simulink model "Discrete_vs_continous"  (R2013a)
settings: Solver=ode45  StartTime=0.0  StopTime=0.1  FixedStep=0.000001  RelTol=1e-3
settings Model: Creator=Max Simmonds  LastModifiedBy=Max Simmonds
settings DebuggingCC: SolverPrmCheckMsg=none

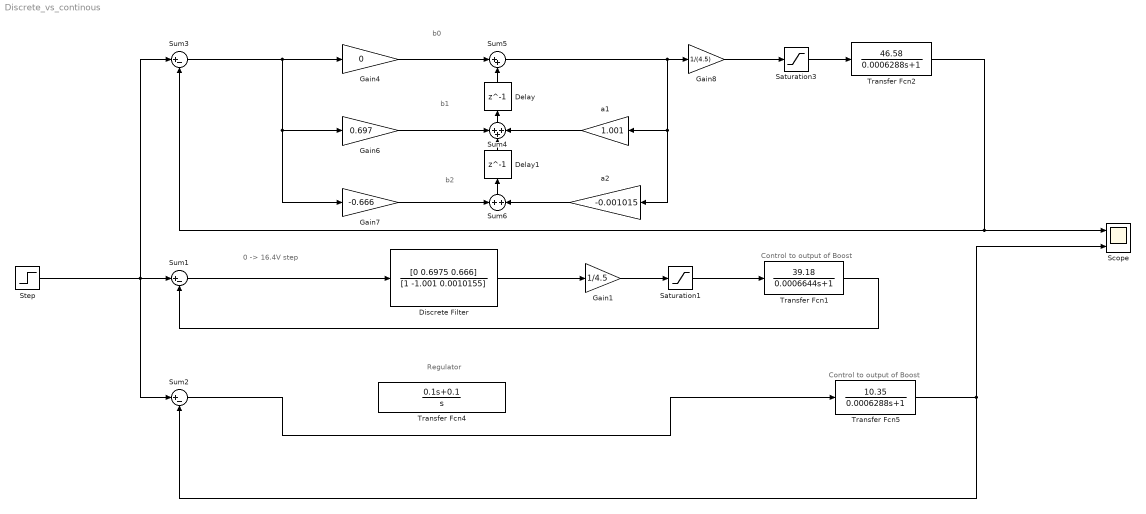
== system Discrete_vs_continous ==
  note: b2
  note: b1
  note: b0
  note: 0 -> 16.4V step
  note: Control to output of Boost
  note: Regulator
  note: Control to output of Boost
  Delay : Delay  DelayLength=1  InitialCondition=0  SampleTime=4e-5
  Delay1 : Delay  DelayLength=1  InitialCondition=0  SampleTime=4e-5
  Discrete Filter : DiscreteFilter  Numerator=[0 0.6975 0.666]  Denominator=[1 -1.001 0.0010155]  SampleTime=4e-5
  Gain1 : Gain  Gain=1/4.5
  Gain4 : Gain  Gain=0  SampleTime=4e-5
  Gain6 : Gain  Gain=0.697  SampleTime=4e-5
  Gain7 : Gain  Gain=-0.666  SampleTime=4e-5
  Gain8 : Gain  Gain=1/(4.5)  SampleTime=4e-5
  Saturation1 : Saturate  UpperLimit=0.9  LowerLimit=0.1
  Saturation3 : Saturate  UpperLimit=0.7  LowerLimit=0.1
  Scope : Scope  NumInputPorts=2
      settings: TimeRange=0.003173749327595482  YMin=15.58~0.334478  YMax=17.22~0.369686
  Step : Step  Time=0.01  Before=0.1  After=16.4  SampleTime=4e-5
  Sum1 : Sum  Inputs=|+-  SampleTime=4e-5
  Sum2 : Sum  Inputs=|+-
  Sum3 : Sum  Inputs=|+-  SampleTime=4e-5
  Sum4 : Sum  Inputs=+++  SampleTime=4e-5
  Sum5 : Sum  Inputs=|++  SampleTime=4e-5
  Sum6 : Sum  SampleTime=4e-5
  Transfer Fcn1 : TransferFcn  Numerator=[39.18]  Denominator=[0.0006644 1]
  Transfer Fcn2 : TransferFcn  Numerator=[46.58]  Denominator=[0.0006288 1]
  Transfer Fcn4 : TransferFcn  Numerator=[0.1 0.1]  Denominator=[1 0]
  Transfer Fcn5 : TransferFcn  Numerator=[10.35]  Denominator=[0.0006288 1]
  a1 : Gain  Gain=1.001  SampleTime=4e-5
  a2 : Gain  Gain=-0.001015  SampleTime=4e-5
  wires:
  Sum2/1 -> Transfer Fcn5/1
  Step/1 -> Sum1/1, Sum3/1, Sum2/1
  Transfer Fcn5/1 -> Sum2/2, Scope/2
  Sum1/1 -> Discrete Filter/1
  Transfer Fcn1/1 -> Sum1/2
  Gain1/1 -> Saturation1/1
  Discrete Filter/1 -> Gain1/1
  Saturation1/1 -> Transfer Fcn1/1
  a1/1 -> Sum4/3
  Gain6/1 -> Sum4/1
  a2/1 -> Sum6/2
  Gain7/1 -> Sum6/1
  Sum3/1 -> Gain7/1, Gain6/1, Gain4/1
  Sum4/1 -> Delay/1
  Delay1/1 -> Sum4/2
  Sum6/1 -> Delay1/1
  Gain8/1 -> Saturation3/1
  Saturation3/1 -> Transfer Fcn2/1
  Sum5/1 -> Gain8/1, a2/1, a1/1
  Delay/1 -> Sum5/2
  Transfer Fcn2/1 -> Scope/1, Sum3/2
  Gain4/1 -> Sum5/1
